simulink model "hdlFrame_adaptiveMedianFilter_MLFB"  (R2022b)
settings: Solver=VariableStepAuto  StartTime=0.0  StopTime=10.0  RelTol=1e-3
undefined symbols (not defined in the file or in its folder): gray, im2gray
settings Model: Creator=kkintali  LastModifiedBy=kkintali
settings SolverCC: MaxZcPerStep=1
settings DebuggingCC: UnconnectedInputMsg=warning  UnconnectedOutputMsg=warning  UnconnectedLineMsg=warning
settings ModelReferenceCC: EnableRefExpFcnMdlSchedulingChecks=on
settings RTWCC: PlatformDefinition=Embedded Code  DLArmComputeVersion=19.05

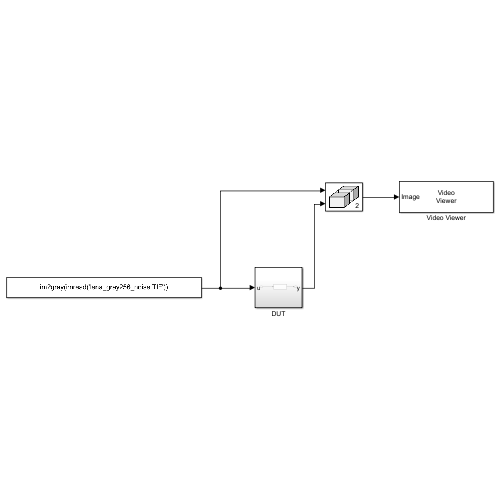
[thumbnail: Simulink's stored preview of the top-level diagram]
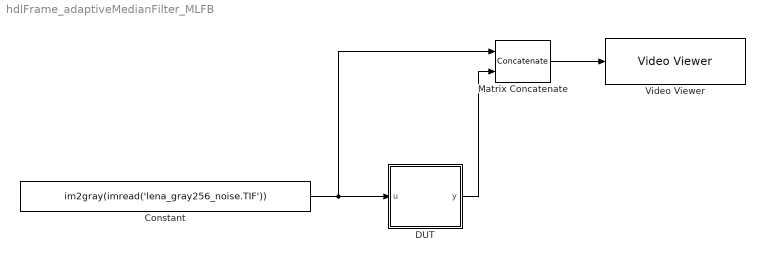
== system hdlFrame_adaptiveMedianFilter_MLFB ==
  Constant : Constant  Value=im2gray(imread('lena_gray256_noise.TIF'))  SampleTime=1
  DUT : Subsystem
  Matrix Concatenate : Concatenate  Mode=Multidimensional array  ConcatenateDimension=2
  Video Viewer : VideoViewer  colormapValue=gray(256)  FigPos=[1575.66666666667 734.666666666667 487.333333333333 288]
  wires:
  Constant/1 -> Matrix Concatenate/1, DUT/1(u)
  DUT/1(y) -> Matrix Concatenate/2
  Matrix Concatenate/1 -> Video Viewer/1

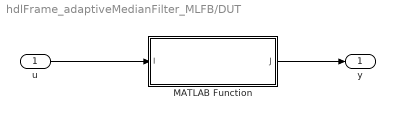
== system hdlFrame_adaptiveMedianFilter_MLFB/DUT ==
  u : Inport
  MATLAB Function : MATLAB Function  TreatAsAtomicUnit=on
  y : Outport
  wires:
  u/1 -> MATLAB Function/1(I)
  MATLAB Function/1(J) -> y/1

== matlab function hdlFrame_adaptiveMedianFilter_MLFB/DUT/MATLAB Function ==
  data: I input; J output
function J = medianFilter3(I) 

J = medianFilter3(I);
